simulink model "deadbeatsimulink"  (R2022b)
settings: Solver=VariableStepAuto  StartTime=0.0  StopTime=30  RelTol=1e-3
values from neighbouring files (symbols this model uses):
  den_dead = [1,-p]    [lab9e10.m]
  disturbio = 0.24    [lab9e10.m]
  q = a*q0    [lab9e10.m]
  R = 1.18    [lab9e10.m]
  T0 = 0.51*1.33    (= 0.6783)    [lab9e10.m]
  tempo_disturbio = 15    [lab9e10.m]
undefined symbols (not defined in the file or in its folder): denPlanta, numPlanta
settings Model: Creator=gusta  LastModifiedBy=gusta

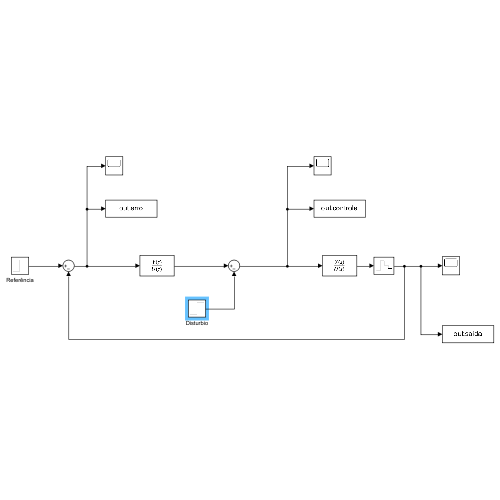
[thumbnail: Simulink's stored preview of the top-level diagram]
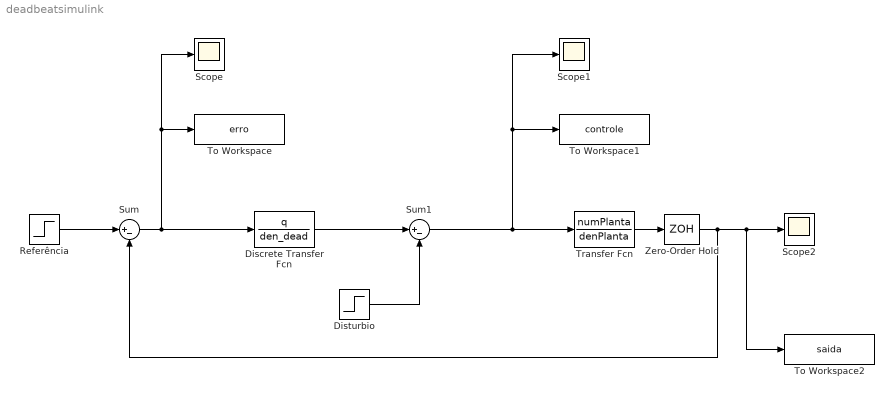
== system deadbeatsimulink ==
  Discrete Transfer Fcn : DiscreteTransferFcn  Numerator=q  Denominator=den_dead  SampleTime=T0
  Disturbio : Step  Time=tempo_disturbio  After=disturbio  SampleTime=0
  Referência : Step  Time=0  After=R  SampleTime=0
  Scope : Scope
  Scope1 : Scope
  Scope2 : Scope
  Sum : Sum  Inputs=|+-
  Sum1 : Sum  Inputs=|+-
  To Workspace : ToWorkspace  VariableName=erro  SaveFormat=Timeseries  SampleTime=-1
  To Workspace1 : ToWorkspace  VariableName=controle  SaveFormat=Timeseries  SampleTime=-1
  To Workspace2 : ToWorkspace  VariableName=saida  SaveFormat=Timeseries  SampleTime=-1
  Transfer Fcn : TransferFcn  Numerator=numPlanta  Denominator=denPlanta
  Zero-Order Hold : ZeroOrderHold  SampleTime=T0
  wires:
  Referência/1 -> Sum/1
  Sum/1 -> Discrete Transfer Fcn/1, Scope/1, To Workspace/1
  Zero-Order Hold/1 -> Sum/2, To Workspace2/1, Scope2/1
  Transfer Fcn/1 -> Zero-Order Hold/1
  Disturbio/1 -> Sum1/2
  Sum1/1 -> Transfer Fcn/1, To Workspace1/1, Scope1/1
  Discrete Transfer Fcn/1 -> Sum1/1
